simulink model "IM_vector_control_v2"  (R2017b)
settings: Solver=FixedStepAuto  StartTime=0.0  StopTime=2  FixedStep=1e-5  MaxStep=1e-4  RelTol=1e-3
values from neighbouring files (symbols this model uses):
  C = [Rs 0 0; 0 Rs 0]    [IM_vector_control_init.m]
  D = [0 -sig*Ls 0; sig*Ls 0 M/Lr]    [IM_vector_control_init.m]
  Lr = 0.274    [IM_vector_control_init.m]
  M = 0.258    [IM_vector_control_init.m]
  p = 2    [IM_vector_control_init.m]
  Tr = Lr/Rr    (= 0.0720105124836)    [IM_vector_control_init.m]
undefined symbols (not defined in the file or in its folder): sigbuilder_block
libraries: powerlib x18, simulink x4, powerlib_meascontrol x1
settings Model: SimulationMode=accelerator  Creator=proso  LastModifiedBy=proso

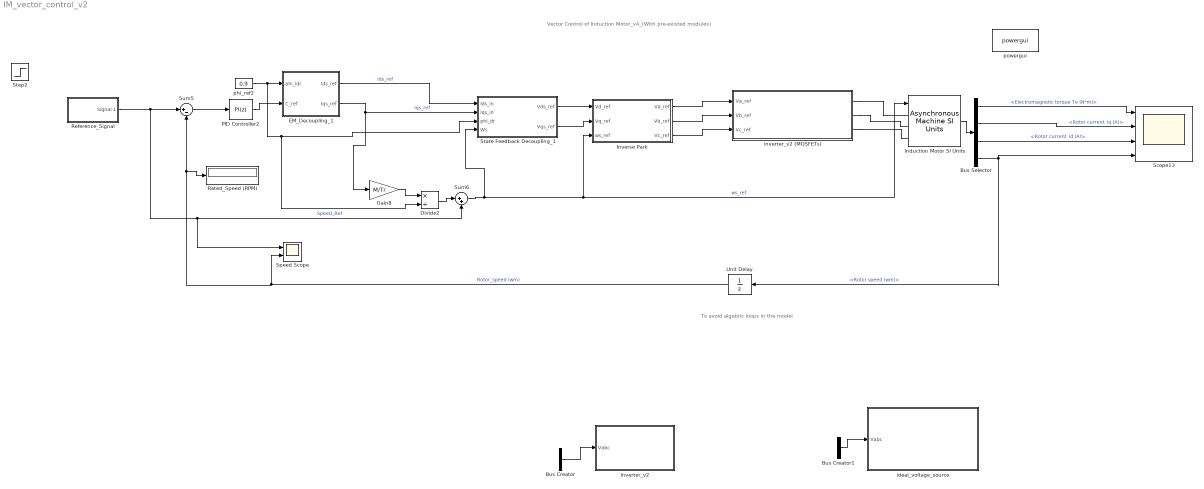
== system IM_vector_control_v2 ==
  note: To avoid algebric loops in the model
  note: Vector Control of Induction Motor_v4_(With pre-existed modules)
  " Inverter_v2" : Subsystem
  Bus Creator : BusCreator  Inputs=3
  Bus Creator1 : BusCreator  Inputs=3
  Bus Selector : BusSelector  OutputSignals="Mechanical.Electromagnetic torque Te (N*m),Rotor measurements.Rotor current  iq (A),Rotor measurements.Rotor current  id (A),Mechanical.Rotor speed (wm)"
  Divide2 : Product  Inputs=*/
  EM_Decoupling_1 : Subsystem
  Gain8 : Gain  Gain=M/Tr
  Induction Motor SI Units : powerlib/Machines/Asynchronous Machine SI Units  RotorType=Squirrel-cage  PresetModel="15:  5.4 HP (4KW)   400 V  50Hz 1430 RPM"  MechanicalLoad=Speed w  ShowDetailedParameters=on  ReferenceFrame=Rotor  Units=SI  MeasurementBus=off  NominalParameters=[4000 400 50]  Stator=[1.405 0.005839]  Rotor=[1.395 0.005839]  Cage1=[0.4155 0.002066]  Cage2=[0.4168 0.0003495]  Lm=0.1722  Mechanical=[0.0131 0.002985 2]  PolePairs=2  InitialConditions=[1 0 0 0 0 0 0 0]  SimulateSaturation=off  Saturation=[14.03593122, 27.81365428, 53.79336849, 72.68890987, 97.98006896, 148.6815601, 215.7428561, 302.9841135, 428.7778367 ; 230, 322, 414, 460, 506, 552, 598, 644, 690]  LoadFlowParameters=1492000  TsPowergui=0  TsBlock=-1  IterativeModel=Trapezoidal non iterative  IterativeDiscreteModel=Trapezoidal non iterative  Pmec=1.492e+006
  Inverse Park : Subsystem
  PID Controller2 : simulink/Continuous/PID Controller  Controller=PI  TimeDomain=Discrete-time  SampleTime=-1  IntegratorMethod=Forward Euler  FilterMethod=Forward Euler  Form=Parallel  UseFilter=on  ControllerParametersSource=internal  P=0.01  I=5  D=1  N=100  InitialConditionSource=internal  InitialConditionForIntegrator=0  InitialConditionForFilter=0  ExternalReset=none  LimitOutput=off  UpperSaturationLimit=inf  LowerSaturationLimit=-inf  LinearizeAsGain=on  AntiWindupMode=none  Kb=1  TrackingMode=off  Kt=1  PParamMin=[]  PParamMax=[]  IParamMin=[]  IParamMax=[]  DParamMin=[]  DParamMax=[]  NParamMin=[]  NParamMax=[]  KbParamMin=[]  KbParamMax=[]  KtParamMin=[]  KtParamMax=[]  POutMin=[]  POutMax=[]  IOutMin=[]  IOutMax=[]  DOutMin=[]  DOutMax=[]  NOutMin=[]  NOutMax=[]  KbOutMin=[]  KbOutMax=[]  KtOutMin=[]  KtOutMax=[]  IntegratorOutMin=[]  IntegratorOutMax=[]  FilterOutMin=[]  FilterOutMax=[]  SumOutMin=[]  SumOutMax=[]  SumI1OutMin=[]  SumI1OutMax=[]  SumI2OutMin=[]  SumI2OutMax=[]  SumI3OutMin=[]  SumI3OutMax=[]  SumDOutMin=[]  SumDOutMax=[]  SaturationOutMin=[]  SaturationOutMax=[]  IntegratorContinuousStateAttributes=''  IntegratorStateMustResolveToSignalObject=off  IntegratorRTWStateStorageClass=Auto  FilterContinuousStateAttributes=''  FilterStateMustResolveToSignalObject=off  FilterRTWStateStorageClass=Auto  DifferentiatorICPrevScaledInput=0  DifferentiatorOutMin=[]  DifferentiatorOutMax=[]  InitialConditionSetting=State (most efficient)  FilterDiffOutCoefMin=[]  FilterDiffOutCoefMax=[]  SumDenOutMin=[]  SumDenOutMax=[]  SumNumOutMin=[]  SumNumOutMax=[]  ReciprocalOutMin=[]  ReciprocalOutMax=[]  DivideOutMin=[]  DivideOutMax=[]  TunerSelectOption=Transfer Function Based (PID Tuner App)
  Rated_Speed (RPM) : Display
  Reference_Signal : Subsystem  Tag=STV Subsys  LoadFcn=sigbuilder_block('load');  StartFcn=sigbuilder_block('start');  StopFcn=sigbuilder_block('stop');  ClipboardFcn=sigbuilder_block('clipboard');  mask(Sigbuilder block){tuvar=[0:10]}
      mask help: Simulink:masks:SigbuilderBlock_MD
      mask init:
      | if ~strcmp(get_param(bdroot(gcbh),'SimulationStatus'),'stopped') tuvar = sigbuilder_block('maskInit'); end
      settings: CopyFcn=sigbuilder_block('copy');  DeleteFcn=sigbuilder_block('delete');  ModelCloseFcn=sigbuilder_block('modelClose');  PreSaveFcn=sigbuilder_block('preSave');  PauseFcn=sigbuilder_block('pause');  ContinueFcn=sigbuilder_block('continue');  NameChangeFcn=sigbuilder_block('namechange');  OpenFcn=sigbuilder_block('open',[250.5 100.5 550.5 359.25 ]);  CloseFcn=sigbuilder_block('close');
      mask Display: plot(0, 0, 100, 100,[2, 2, 32, 32, 2], [68, 8, 8, 68, 68],[32, 2], [38, 38], [32, 19, 2],[53, 60, 44], [32, 17, 17, 2],[16, 16, 31, 31]);txt = getActiveGroup(gcbh);text(2, 100, txt,'verticalAlignment', 'top');
  Scope13 : Scope  NumInputPorts=4
  Speed Scope : Scope  NumInputPorts=2
  State Feedback Decoupling_1 : Subsystem
  Step2 : Step  Time=0.5  After=1000  SampleTime=0
  Sum5 : Sum  Inputs=|+-
  Sum6 : Sum  Inputs=|++
  Unit Delay : UnitDelay  SampleTime=-1
  ideal_voltage_source : Subsystem  VariantControl=variantPwm == enumPwm.behavior
  inverter_v2 (MOSFETs) : Subsystem
  phi_ref2 : Constant  Value=0.9
  powergui : powerlib/powergui  Priority=1  SimulationMode=Discrete  SampleTime=1e-5  frequency=60  Iterations=50  frequencyindice=0  Pbase=100e6  ErrMax=1e-4  UnitsV=kV  UnitsW=MW  buscounter=0  FunctionMessages=off  echomessages=off  EnableUseOfTLC=off  CurrentSourceSwitches=off  DisableSnubberDevices=off  DisableRonSwitches=off  DisableVfSwitches=off  DisplayEquations=off  SolverType=Tustin/Backward Euler (TBE)  Interpol=off  ExternalGateDelay=off  methode=off  Ts=100  x0status=blocks  SPID=off  SwTol=0  HookPort=off  RestoreLinks=warning  ResistiveCurrentMeasurement=off  Frange=[0:2:500]  Ylog=off  Xlog=on  ShowGrid=off  save=off  variable=ZData  structure=0  ZoomFFT=off  StartTime=0.0  cycles=1  DisplayStyle=1  fundamental=60  FreqAxis=off  MaxFrequency=1000  frequencyindicesteady=1  RmsSteady=1  display=off
  wires:
  Sum6/1 -> Induction Motor SI Units/1, Inverse Park/3(ws_ref), State Feedback Decoupling_1/4(Ws)  "ws_ref"
  Bus Selector/2 -> Scope13/2  "<Rotor current  iq (A)>"
  Induction Motor SI Units/1 -> Bus Selector/1
  State Feedback Decoupling_1/1(Vds_ref) -> Inverse Park/1(Vd_ref)
  Gain8/1 -> Divide2/1
  Sum5/1 -> PID Controller2/1
  Divide2/1 -> Sum6/1
  EM_Decoupling_1/1(Ids_ref) -> State Feedback Decoupling_1/1(Ids_in)  "ids_ref"
  EM_Decoupling_1/2(Iqs_ref) -> State Feedback Decoupling_1/2(Iqs_in), Gain8/1  "iqs_ref"
  PID Controller2/1 -> EM_Decoupling_1/2(C_ref)
  Reference_Signal/1(Signal 1) -> Speed Scope/1, Sum6/2, Sum5/1  "Speed_Ref"
  Bus Selector/1 -> Scope13/1  "<Electromagnetic torque Te (N*m)>"
  phi_ref2/1 -> State Feedback Decoupling_1/3(phi_dr), Divide2/2, EM_Decoupling_1/1(phi_idr)
  Bus Selector/3 -> Scope13/3  "<Rotor current  id (A)>"
  Bus Selector/4 -> Scope13/4, Unit Delay/1  "<Rotor speed (wm)>"
  State Feedback Decoupling_1/2(Vqs_ref) -> Inverse Park/2(Vq_ref)
  ? -> Bus Creator/1
  ? -> Bus Creator/2
  Bus Creator/1 -> " Inverter_v2"/1(Vabc)
  ? -> Bus Creator/3
  Inverse Park/1(Va_ref) -> inverter_v2 (MOSFETs)/1(Va_ref)
  Inverse Park/2(Vb_ref) -> inverter_v2 (MOSFETs)/2(Vb_ref)
  Inverse Park/3(Vc_ref) -> inverter_v2 (MOSFETs)/3(Vc_ref)
  Bus Creator1/1 -> ideal_voltage_source/1(Vabc)
  ? -> Bus Creator1/2
  ? -> Bus Creator1/1
  ? -> Bus Creator1/3
  Unit Delay/1 -> Rated_Speed (RPM)/1, Sum5/2, Speed Scope/2  "Rotor_speed (wm)"
  connections:
  inverter_v2 (MOSFETs)/RConn2 -- Induction Motor SI Units/LConn2
  inverter_v2 (MOSFETs)/RConn1 -- Induction Motor SI Units/LConn1
  inverter_v2 (MOSFETs)/RConn3 -- Induction Motor SI Units/LConn3

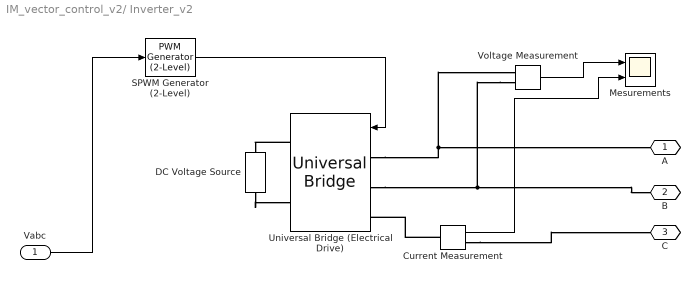
== system IM_vector_control_v2/ Inverter_v2 ==
  Vabc : Inport
  Current Measurement : powerlib/Measurements/Current Measurement  PhasorSimulation=off  OutputType=Complex  PSBequivalent=0
  DC Voltage Source : powerlib/Electrical Sources/DC Voltage Source  Amplitude=660  Measurements=None
  Mesurements : Scope  NumInputPorts=2
  SPWM Generator (2-Level) : powerlib_meascontrol/Pulse & Signal Generators/PWM Generator (2-Level)  ModulatorType=Three-phase bridge (6 pulses)  ModulatorMode=Unsynchronized  Fc=50  Pc=90  nF=27  MinMax="[ -1  1 ]"  SamplingTechnique=Natural  ModulatingSignals=off  m=0.8  Freq=60  Phase=0  Ts=0  ShowCarrierOutport=off
      settings: SourceProductName=Simscape Power Systems
  Universal Bridge (Electrical Drive) : powerlib/Power Electronics/Universal Bridge  Arms=3  SnubberResistance=1e5  SnubberCapacitance=inf  Device=IGBT / Diodes  Ron=1e-3  Lon=0  ForwardVoltages="[  0  0  ]"  ForwardVoltage=0  GTOparameters=[ 10e-6 , 20e-6 ]  IGBTparameters=[ 1e-6 , 2e-6 ]  Measurements=None  Measurements_2=None  converterType=Rectifier
  Voltage Measurement : powerlib/Measurements/Voltage Measurement  PhasorSimulation=off  OutputType=Complex  PSBequivalent=0
  A : PMIOPort  Port=1  Side=Right
  B : PMIOPort  Port=2  Side=Right
  C : PMIOPort  Port=3  Side=Right
  wires:
  SPWM Generator (2-Level)/1 -> Universal Bridge (Electrical Drive)/1
  Vabc/1 -> SPWM Generator (2-Level)/1
  Voltage Measurement/1 -> Mesurements/1
  Current Measurement/1 -> Mesurements/2
  connections:
  Universal Bridge (Electrical Drive)/RConn1 -- DC Voltage Source/RConn1
  DC Voltage Source/LConn1 -- Universal Bridge (Electrical Drive)/RConn2
  Current Measurement/LConn1 -- Universal Bridge (Electrical Drive)/LConn3
  Universal Bridge (Electrical Drive)/LConn1 -- Voltage Measurement/LConn1 -- A/RConn1
  Voltage Measurement/LConn2 -- Universal Bridge (Electrical Drive)/LConn2 -- B/RConn1
  Current Measurement/RConn1 -- C/RConn1

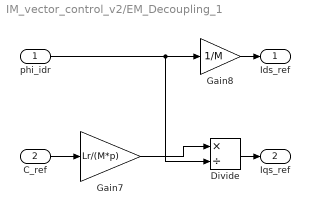
== system IM_vector_control_v2/EM_Decoupling_1 ==
  phi_idr : Inport
  C_ref : Inport  Port=2
  Divide : Product  Inputs=*/
  Gain7 : Gain  Gain=Lr/(M*p)
  Gain8 : Gain  Gain=1/M
  Ids_ref : Outport
  Iqs_ref : Outport  Port=2
  wires:
  Gain8/1 -> Ids_ref/1
  Divide/1 -> Iqs_ref/1
  C_ref/1 -> Gain7/1
  Gain7/1 -> Divide/1
  phi_idr/1 -> Divide/2, Gain8/1

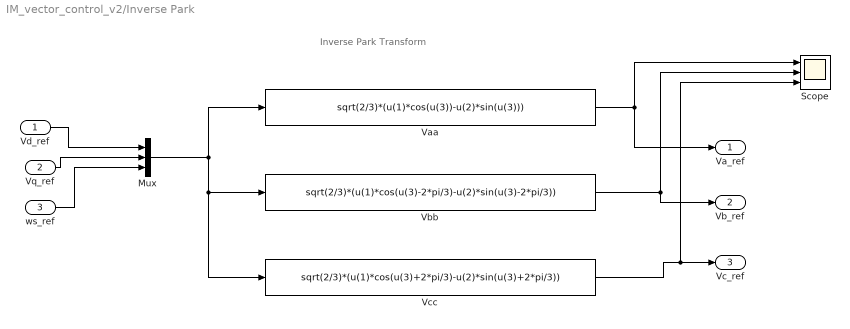
== system IM_vector_control_v2/Inverse Park ==
  note: Inverse Park Transform
  Vd_ref : Inport
  Vq_ref : Inport  Port=2
  ws_ref : Inport  Port=3
  Mux : Mux  Inputs=3
  Scope : Scope  NumInputPorts=3
  Vaa : Fcn  Expr=sqrt(2/3)*(u(1)*cos(u(3))-u(2)*sin(u(3)))
  Vbb : Fcn  Expr=sqrt(2/3)*(u(1)*cos(u(3)-2*pi/3)-u(2)*sin(u(3)-2*pi/3))
  Vcc : Fcn  Expr=sqrt(2/3)*(u(1)*cos(u(3)+2*pi/3)-u(2)*sin(u(3)+2*pi/3))
  Va_ref : Outport
  Vb_ref : Outport  Port=2
  Vc_ref : Outport  Port=3
  wires:
  Vd_ref/1 -> Mux/1
  Vq_ref/1 -> Mux/2
  ws_ref/1 -> Mux/3
  Mux/1 -> Vcc/1, Vbb/1, Vaa/1
  Vaa/1 -> Va_ref/1, Scope/1
  Vbb/1 -> Vb_ref/1, Scope/2
  Vcc/1 -> Scope/3, Vc_ref/1

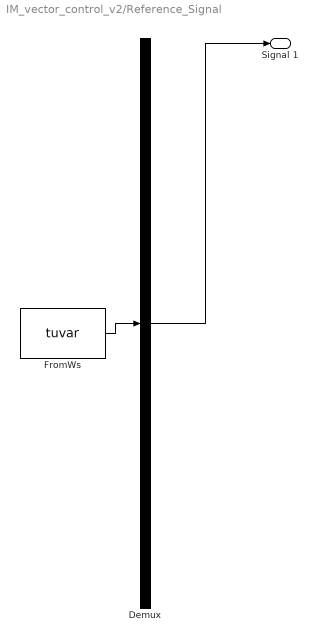
== system IM_vector_control_v2/Reference_Signal ==
  Demux : Demux  Tag=STV Demux  Outputs=1
  FromWs : FromWorkspace  Tag=STV FromWs  VariableName=tuvar  SampleTime=0
      SigBuilderData=|
      | common.afterFinalStr = 'Extrapolate'
      | common.sampleTime = 0
      | dataSet.timeRange = [0 2]
      | dataSet.name = 'Group 1'
      | sbobj.Groups.Name = 'Group 1'
      | sbobj.Groups.Signals.Name = 'Signal 1'
      | sbobj.Groups.Signals.XData = [0 0.5 0.5 0.74 0.74 1.16 1.16 1.715 1.715 2]
      | sbobj.Groups.Signals.YData = [0 0 500 500 800 800 1280 1280 790 790]
      | sbobj.Groups.TimeRange = [0 2]
  Signal 1 : Outport  Tag=STV Outport
  wires:
  Demux/1 -> Signal 1/1
  FromWs/1 -> Demux/1

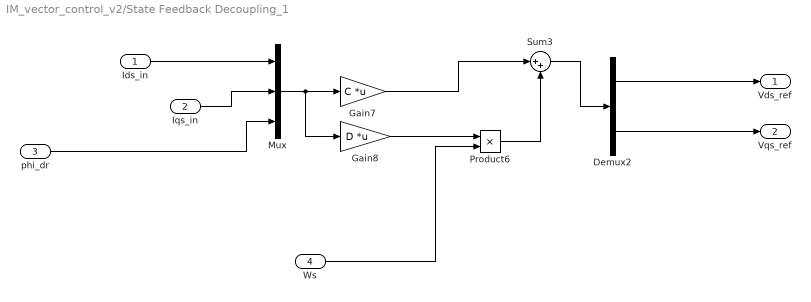
== system IM_vector_control_v2/State Feedback Decoupling_1 ==
  Ids_in : Inport
  Iqs_in : Inport  Port=2
  phi_dr : Inport  Port=3
  Ws : Inport  Port=4
  Demux2 : Demux  Outputs=2
  Gain7 : Gain  Gain=C  Multiplication=Matrix(K*u)
  Gain8 : Gain  Gain=D  Multiplication=Matrix(K*u)
  Mux : Mux  Inputs=3
  Product6 : Product
  Sum3 : Sum  Inputs=|++
  Vds_ref : Outport
  Vqs_ref : Outport  Port=2
  wires:
  Iqs_in/1 -> Mux/2
  phi_dr/1 -> Mux/3
  Ids_in/1 -> Mux/1
  Mux/1 -> Gain8/1, Gain7/1
  Ws/1 -> Product6/2
  Gain8/1 -> Product6/1
  Sum3/1 -> Demux2/1
  Demux2/2 -> Vqs_ref/1
  Demux2/1 -> Vds_ref/1
  Gain7/1 -> Sum3/1
  Product6/1 -> Sum3/2

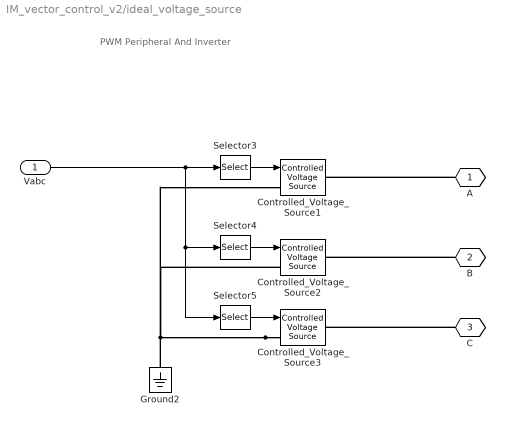
== system IM_vector_control_v2/ideal_voltage_source ==
  note: PWM Peripheral And Inverter
  Vabc : Inport
  Controlled_Voltage_Source1 : powerlib/Electrical Sources/Controlled Voltage Source  Initialize=off  Source_Type=DC  Amplitude=12  Phase=0  Frequency=0  Measurements=None
  Controlled_Voltage_Source2 : powerlib/Electrical Sources/Controlled Voltage Source  Initialize=off  Source_Type=DC  Amplitude=12  Phase=0  Frequency=0  Measurements=None
  Controlled_Voltage_Source3 : powerlib/Electrical Sources/Controlled Voltage Source  Initialize=off  Source_Type=DC  Amplitude=12  Phase=0  Frequency=0  Measurements=None
  Ground2 : powerlib/Elements/Ground  LConnTagsString=a
  Selector3 : Selector  InputPortWidth=3  IndexOptions=Index vector (dialog)  Indices=[1]  OutputSizes=1
  Selector4 : Selector  InputPortWidth=3  IndexOptions=Index vector (dialog)  Indices=2  OutputSizes=1
  Selector5 : Selector  InputPortWidth=3  IndexOptions=Index vector (dialog)  Indices=3  OutputSizes=1
  A : PMIOPort  Tag=PMCPort  Port=1  Side=Right
  B : PMIOPort  Tag=PMCPort  Port=2  Side=Right
  C : PMIOPort  Tag=PMCPort  Port=3  Side=Right
  wires:
  Vabc/1 -> Selector4/1, Selector5/1, Selector3/1
  Selector5/1 -> Controlled_Voltage_Source3/1
  Selector4/1 -> Controlled_Voltage_Source2/1
  Selector3/1 -> Controlled_Voltage_Source1/1
  connections:
  C/RConn1 -- Controlled_Voltage_Source3/RConn1
  B/RConn1 -- Controlled_Voltage_Source2/RConn1
  A/RConn1 -- Controlled_Voltage_Source1/RConn1
  Controlled_Voltage_Source3/LConn1 -- Controlled_Voltage_Source1/LConn1 -- Controlled_Voltage_Source2/LConn1 -- Ground2/LConn1

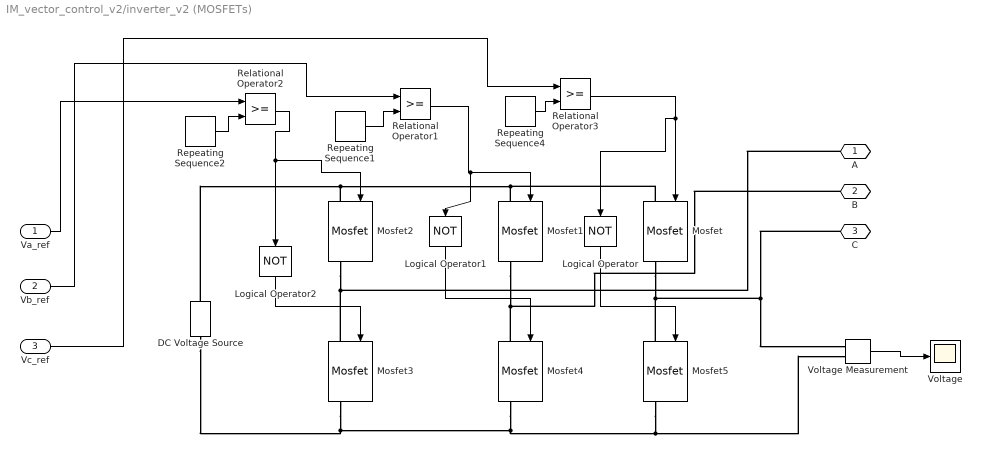
== system IM_vector_control_v2/inverter_v2 (MOSFETs) ==
  Va_ref : Inport
  Vb_ref : Inport  Port=2
  Vc_ref : Inport  Port=3
  DC Voltage Source : powerlib/Electrical Sources/DC Voltage Source  Amplitude=660  Measurements=None
  Logical Operator : Logic  Operator=NOT  AllPortsSameDT=off  OutDataTypeStr=boolean
  Logical Operator1 : Logic  Operator=NOT  AllPortsSameDT=off  OutDataTypeStr=boolean
  Logical Operator2 : Logic  Operator=NOT  AllPortsSameDT=off  OutDataTypeStr=boolean
  Mosfet{,1..5} (6 alike) : powerlib/Power Electronics/Mosfet  Ron=0.1  Lon=0  Rd=0.01  Vfd=0  IC=0  Rs=1e5  Cs=inf  Measurements=on
  Relational Operator1 : RelationalOperator  OutDataTypeStr=boolean  RndMeth=Simplest
  Relational Operator2 : RelationalOperator  OutDataTypeStr=boolean  RndMeth=Simplest
  Relational Operator3 : RelationalOperator  OutDataTypeStr=boolean  RndMeth=Simplest
  Repeating Sequence1 : simulink/Sources/Repeating Sequence  rep_seq_t="[0 (1/5000)/4  (1/5000)/2 (3/5000)/4 1/5000]"  rep_seq_y=[0 1 0 -1 0]
  Repeating Sequence2 : simulink/Sources/Repeating Sequence  rep_seq_t="[0 (1/5000)/4  (1/5000)/2 (3/5000)/4 1/5000]"  rep_seq_y=[0 1 0 -1 0]
  Repeating Sequence4 : simulink/Sources/Repeating Sequence  rep_seq_t="[0 (1/5000)/4  (1/5000)/2 (3/5000)/4 1/5000]"  rep_seq_y=[0 1 0 -1 0]
  Voltage : Scope
  Voltage Measurement : powerlib/Measurements/Voltage Measurement  PhasorSimulation=off  OutputType=Complex  PSBequivalent=0
  A : PMIOPort  Port=1  Side=Right
  B : PMIOPort  Port=2  Side=Right
  C : PMIOPort  Port=3  Side=Right
  wires:
  Relational Operator1/1 -> Mosfet1/1, Logical Operator1/1
  Vc_ref/1 -> Relational Operator3/1
  Logical Operator2/1 -> Mosfet3/1
  Va_ref/1 -> Relational Operator2/1
  Repeating Sequence4/1 -> Relational Operator3/2
  Repeating Sequence2/1 -> Relational Operator2/2
  Repeating Sequence1/1 -> Relational Operator1/2
  Relational Operator3/1 -> Mosfet/1, Logical Operator/1
  Relational Operator2/1 -> Mosfet2/1, Logical Operator2/1
  Vb_ref/1 -> Relational Operator1/1
  Logical Operator/1 -> Mosfet5/1
  Logical Operator1/1 -> Mosfet4/1
  Voltage Measurement/1 -> Voltage/1
  connections:
  Mosfet/LConn1 -- Mosfet1/LConn1 -- DC Voltage Source/RConn1 -- Mosfet2/LConn1
  Mosfet/RConn1 -- Voltage Measurement/LConn1 -- C/RConn1 -- Mosfet5/LConn1
  Mosfet2/RConn1 -- A/RConn1 -- Mosfet3/LConn1
  Mosfet5/RConn1 -- DC Voltage Source/LConn1 -- Mosfet3/RConn1 -- Mosfet4/RConn1 -- Voltage Measurement/LConn2
  Mosfet1/RConn1 -- B/RConn1 -- Mosfet4/LConn1
